simulink model "diagbloque3prueba"  (R2019b)
settings: Solver=VariableStepAuto  StartTime=0.0  StopTime=10  RelTol=1e-3  EnableMultiTasking=on
values from neighbouring files (symbols this model uses):
  ba = 0.001    [TPpelotita.m]
  bp = 1.59    [TPpelotita.m]
  m = 0.0585    [TPpelotita.m]
  r = 0.063/2    (= 0.0315)    [TPpelotita.m]
  v0y = -100    [TPpelotita.m]
  y0 = 1.5    [TPpelotita.m]
undefined symbols (not defined in the file or in its folder): k
libraries: simulink_extras x1
settings Model: Creator=Paula  LastModifiedBy=Fer
settings DataIOCC: ReturnWorkspaceOutputs=off
settings OptimizationCC: LifeSpan=inf
settings DebuggingCC: SFUnexpectedBacktrackingDiag=warning  SFNoUnconditionalDefaultTransitionDiag=warning  ArithmeticOperatorsInVariantConditions=warning
settings SFSimCC: SimUseLocalCustomCode=off  CustomCodeUndefinedFunction=UseInterfaceOnly
settings RTWCC: RTWUseLocalCustomCode=off
settings CodeAppCC: StateflowObjectComments=on
settings GRTTargetCC: TargetLangStandard=C89/C90 (ANSI)  GeneratePreprocessorConditionals=Disable all
settings ConfigComp: CovMetricSettings=dw  CovHtmlReporting=on  CovSaveCumulativeToWorkspaceVar=on  CovSaveSingleToWorkspaceVar=on  CovExternalEMLEnable=off

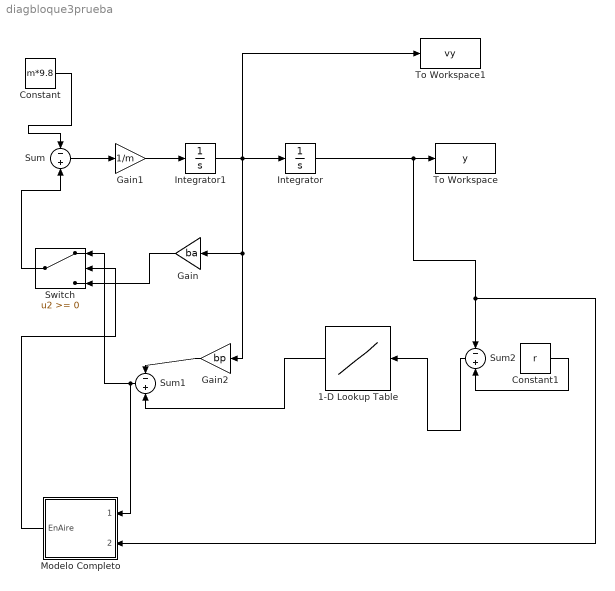
== system diagbloque3prueba ==
  1-D Lookup Table : Lookup_n-D  NumberOfTableDimensions=1  BreakpointsForDimension1=[0,0.000152979,0.000299869,0.000439218,0.000573908,0.000701165,0.000827118,0.000954278,0.001083536,0.001209584,0.001340158,0.001478477,0.00161775,0.001752221,0.001887395,0.002024889]  Table=[0,0.0686,0.4214,1.029,1.8424,3.0282,4.4492,6.0564,7.84,10.241,12.74,14.798,16.905,19.6392,22.344,24.843]  InternalRulePriority=Speed  RndMeth=Simplest  InputSameDT=on
  Constant : Constant  Value=m*9.8
  Constant1 : Constant  Value=r
  Gain : Gain  Gain=ba
  Gain1 : Gain  Gain=1/m
  Gain2 : Gain  Gain=bp
  Integrator : Integrator  InitialCondition=y0
  Integrator1 : Integrator  InitialCondition=v0y
  Modelo Completo : Subsystem  mask{r=r, b=bp, k=k, yp0=y0-r}
      mask prompts: r "Radio"; b "Coef. friccion"; k "Coef. elasticidad"; yp0 "Posicion Inicial pto. inferior"
      mask help: La salida 'EnAire' es 1 inicialmente. 'EnAire' cambia a 0 cuando una variable interna que representa la posicion del punto inferior de la pelota llega a 0 con tendencia descendente. Cuando 'EnAire' es 0, cambiarÃ¡ a 1 cuando 'Fnormal' llegue a 0 con tendencia descendente.
  Sum : Sum  Inputs=-+
  Sum1 : Sum  Inputs=-+
  Sum2 : Sum  Inputs=-+
  Switch : Switch
  To Workspace : ToWorkspace  VariableName=y  SaveFormat=Structure With Time  SampleTime=0.01
  To Workspace1 : ToWorkspace  VariableName=vy  SaveFormat=Structure With Time  SampleTime=0.01
  wires:
  Switch/1 -> Sum/2
  Gain1/1 -> Integrator1/1
  Integrator1/1 -> To Workspace1/1, Gain2/1, Gain/1, Integrator/1
  Gain2/1 -> Sum1/1
  1-D Lookup Table/1 -> Sum1/2
  Constant1/1 -> Sum2/2
  Sum2/1 -> 1-D Lookup Table/1
  Integrator/1 -> Modelo Completo/2(Posicion CM), Sum2/1, To Workspace/1
  Sum/1 -> Gain1/1
  Constant/1 -> Sum/1
  Sum1/1 -> Modelo Completo/1(Fnormal), Switch/1
  Gain/1 -> Switch/3
  Modelo Completo/1(EnAire) -> Switch/2

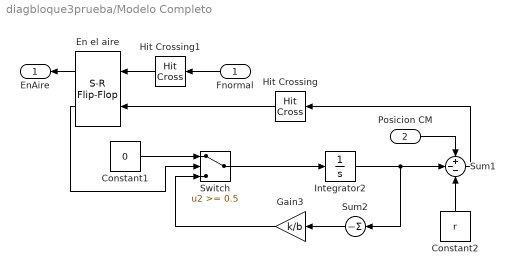
== system diagbloque3prueba/Modelo Completo ==
  Fnormal : Inport
  Posicion CM : Inport  Port=2
  Constant1 : Constant  Value=0
  Constant2 : Constant  Value=r
  En el aire : simulink_extras/Flip Flops/S-R Flip-Flop  initial_condition=1
  Gain3 : Gain  Gain=k/b
  Hit Crossing : HitCross  HitCrossingDirection=falling
  Hit Crossing1 : HitCross  HitCrossingDirection=falling
  Integrator2 : Integrator  InitialCondition=yp0
  Sum1 : Sum  Inputs=+--
  Sum2 : Sum  Inputs=-
  Switch : Switch  Threshold=0.5
  EnAire : Outport
  wires:
  En el aire/2 -> Switch/2
  Constant1/1 -> Switch/1
  Gain3/1 -> Switch/3
  Switch/1 -> Integrator2/1
  Sum2/1 -> Gain3/1
  Integrator2/1 -> Sum2/1, Sum1/2
  En el aire/1 -> EnAire/1
  Fnormal/1 -> Hit Crossing1/1
  Hit Crossing/1 -> En el aire/2
  Hit Crossing1/1 -> En el aire/1
  Constant2/1 -> Sum1/3
  Posicion CM/1 -> Sum1/1
  Sum1/1 -> Hit Crossing/1
